simulink model "verify_pressure_drop_quadratic_fitted_data_mdl"  (R2016b)
settings: Solver=VariableStepDiscrete  StartTime=0  StopTime=200  MaxStep=1  RelTol=1e-3  EnableMultiTasking=on
InitFcn:
  | acol = 2.5;
libraries: simulink x1, carnot x1
settings Model: Creator=drhf  LastModifiedBy=User
settings DataIOCC: SaveFormat=Array  SignalLoggingSaveFormat=ModelDataLogs
settings OptimizationCC: ExpressionDepthLimit=2147483647  LifeSpan=inf
settings DebuggingCC: UnderspecifiedInitializationDetection=Classic  MergeDetectMultiDrivingBlocksExec=none  SolverPrmCheckMsg=warning  FcnCallInpInsideContextMsg=warning  StateNameClashWarn=warning  SFUnexpectedBacktrackingDiag=warning  SFNoUnconditionalDefaultTransitionDiag=warning  SFExecutionAtInitializationDiag=none
settings HardwareCC: ProdBitPerPointer=32  ProdBitPerSizeT=32  ProdBitPerPtrDiffT=32  ProdLargestAtomicFloat=None  ProdIntDivRoundTo=Undefined  ProdEndianess=Unspecified  ProdWordSize=32  ProdHWDeviceType=32-bit Generic
settings ModelReferenceCC: PropagateSignalLabelsOutOfModel=off
settings GRTTargetCC: TargetLangStandard=C89/C90 (ANSI)  GeneratePreprocessorConditionals=Disable all  CombineOutputUpdateFcns=off  GRTInterface=on
settings ConfigComp: CovMetricSettings=dw  CovHtmlReporting=on  CovSaveCumulativeToWorkspaceVar=on  CovSaveSingleToWorkspaceVar=on  CovExternalEMLEnable=off

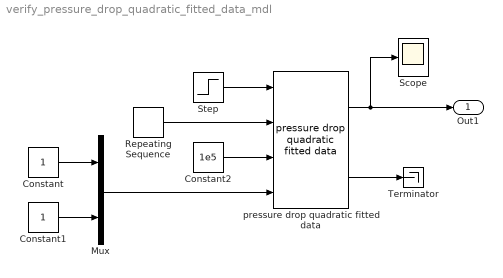
== system verify_pressure_drop_quadratic_fitted_data_mdl ==
  Constant : Constant
  Constant1 : Constant
  Constant2 : Constant  Value=1e5
  Mux : Mux  Inputs=2
  Repeating Sequence : simulink/Sources/Repeating Sequence  rep_seq_t=[0 50 100]  rep_seq_y=[100/3600 500/3600 100/3600]
  Scope : Scope
  Step : Step  Time=100  Before=20  After=40  SampleTime=0
  Terminator : Terminator
  pressure drop quadratic fitted data : carnot/Source/Solar_Thermal/PressureDropCollector/pressure drop quadratic fitted data  b=0.006201*3.6e4  a=0.000096*1.296e9  aonecol=1.96  acol=acol
  Out1 : Outport
  wires:
  pressure drop quadratic fitted data/1 -> Out1/1, Scope/1
  pressure drop quadratic fitted data/2 -> Terminator/1
  Mux/1 -> pressure drop quadratic fitted data/4
  Constant/1 -> Mux/1
  Constant1/1 -> Mux/2
  Constant2/1 -> pressure drop quadratic fitted data/3
  Repeating Sequence/1 -> pressure drop quadratic fitted data/2
  Step/1 -> pressure drop quadratic fitted data/1
